simulink model "simhope"  (R2015b)
settings: Solver=VariableStepAuto  StartTime=0.0  StopTime=10.0  RelTol=1e-3
settings Model: Creator=29118  LastModifiedBy=朱明菲

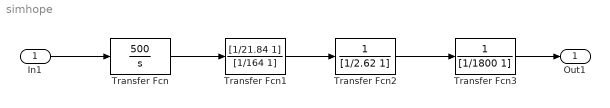
== system simhope ==
  In1 : Inport
  Transfer Fcn : TransferFcn  Numerator=[500]  Denominator=[1 0]
  Transfer Fcn1 : TransferFcn  Numerator=[1/21.84 1]  Denominator=[1/164 1]
  Transfer Fcn2 : TransferFcn  Denominator=[1/2.62 1]
  Transfer Fcn3 : TransferFcn  Denominator=[1/1800 1]
  Out1 : Outport
  wires:
  In1/1 -> Transfer Fcn/1
  Transfer Fcn/1 -> Transfer Fcn1/1
  Transfer Fcn1/1 -> Transfer Fcn2/1
  Transfer Fcn2/1 -> Transfer Fcn3/1
  Transfer Fcn3/1 -> Out1/1
